simulink model "composition"  (R2024a)
settings: Solver=FixedStepDiscrete  StartTime=0.0  StopTime=10.0  RelTol=1e-3  EnableMultiTasking=on
undefined symbols (not defined in the file): D1, P
libraries: autosarlibdem x1, autosarlibnvm x1
settings Model: Creator=buiqu  LastModifiedBy=buiqu
settings SolverCC: AlgebraicLoopSolver=TrustRegion  AutoInsertRateTranBlk=on  InsertRTBMode=Never (minimum delay)  MaxZcPerStep=1
settings OptimizationCC: DefaultParameterBehavior=Inlined  EnhancedBackFolding=on  PassReuseOutputArgsAs=Individual arguments  ZeroExternalMemoryAtStartup=off  ZeroInternalMemoryAtStartup=off  OptimizeBlockOrder=speed  DifferentSizesBufferReuse=on  OptimizationCustomize=off  EfficientTunableParamExpr=on
settings DebuggingCC: MultiTaskDSMMsg=none  MultiTaskRateTransMsg=warning  ParameterTunabilityLossMsg=error  UnconnectedLineMsg=warning
settings ModelReferenceCC: EnableRefExpFcnMdlSchedulingChecks=on
settings SFSimCC: MATLABDynamicMemAlloc=off
settings RTWCC: Description=AUTOSAR  SystemTargetFile=autosar.tlc  GenCodeOnly=on  TemplateMakefile=ert_default_tmf  IncludeHyperlinkInReport=on  DataTypeReplacement=CDataTypesFixedWidth  GPUComputeCapability=3.5  DLArmComputeVersion=19.05
settings CodeAppCC: ForceParamTrailComments=on  IgnoreCustomStorageClasses=off  OperatorAnnotations=on  SimulinkDataObjDesc=on  SFDataObjDesc=on  InsertBlockDesc=on
settings STFCustomTargetCC: MultiwordLength=256  ParMdlRefBuildCompliant=on  CompOptLevelCompliant=on  IncludeMdlTerminateFcn=off  CombineOutputUpdateFcns=on  SuppressErrorStatus=on  ERTCustomFileBanners=on  SupportNonFinite=off  SupportComplex=off  SupportContinuousTime=off  SupportNonInlinedSFcns=off  RemoveResetFunc=on  MATLABClassNameForMDSCustomization=Simulink.SoftwareTarget.ERTCustomization  AutosarCompliant=on  GRTInterface=off  LookupTableObjectStructAxisOrder=2,1,3,4,...  LUTObjectStructOrderEvenSpacing=Size,Table,Breakpoints  SystemTargetFile=autosar.tlc
settings ERTTargetCC: TargetLangStandard=C99 (ISO)  ConcurrentExecutionCompliant=off  IncludeMdlTerminateFcn=off  SuppressErrorStatus=on  SupportNonFinite=off  SupportComplex=off  ModelStepFunctionPrototypeControlCompliant=off  CPPClassGenCompliant=off  AutosarCompliant=on  LookupTableObjectStructAxisOrder=2,1,3,4,...  LUTObjectStructOrderEvenSpacing=Size,Table,Breakpoints  InlinedParameterPlacement=NonHierarchical  ERTCustomFileTemplate=example_file_process.tlc  BooleanTrueId=TRUE  BooleanFalseId=FALSE

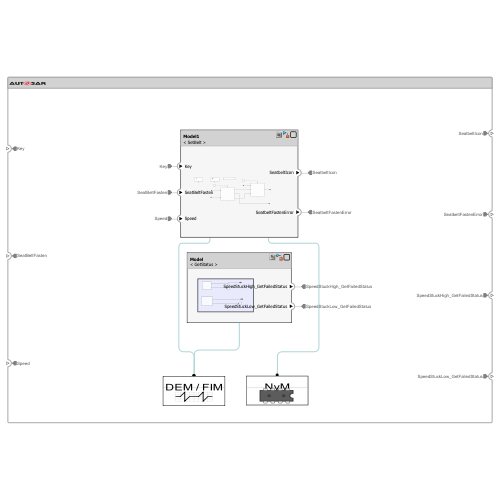
[thumbnail: Simulink's stored preview of the top-level diagram]
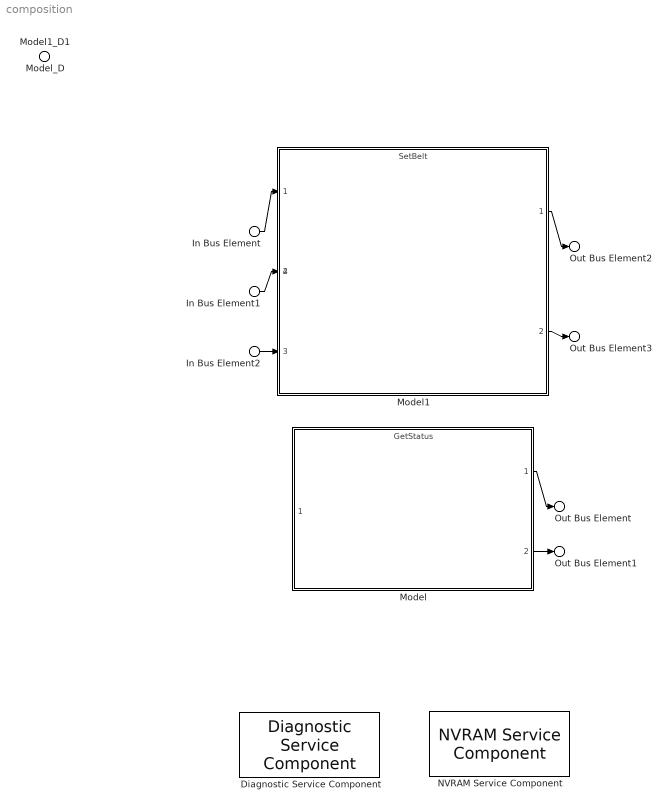
== system composition ==
  In Bus Element : Inport  PortName=Key
  In Bus Element1 : Inport  Port=2  PortName=SeatBeltFasten
  In Bus Element2 : Inport  Port=3  PortName=Speed
  Model_D : Inport  Port=4  OutputFunctionCall=on
  Model1_D1 : Inport  Port=5  OutputFunctionCall=on
  Diagnostic Service Component : autosarlibdem/Diagnostic Service Component  ClientPortNames={'SpeedStuckHigh', 'SpeedStuckLow'}  ClientPortPortDefinedArguments={'1', '2'}  MaxEventId=2  MaxFID=1  DemDebounceCounterIncrementStepSize=1  DemDebounceCounterDecrementStepSize=1  DemDebounceCounterFailedThreshold=2  DemDebounceCounterPassedThreshold=-1  InhibitionMatrix=[0 0;0 0]  EnableConditionIndexes=zeros(257,'uint8')  StorageConditionIndexes=zeros(257,'uint8')
  Model : ModelReference  ModelNameDialog=GetStatus  SimulationMode=Normal  ScheduleRates=on  CachedPortDiscreteRates=[-1]  ModelEventPortInfo=P:D1[-1][0][0]  CodeInterface=Top model  ModelReferenceVersion=1.12
      settings: PortSchema="{\"entries\":[{\"content\":{\"headerSize\":38,\"margin\":15,\"minimumSpacing\":25,\"sides\":[{\"content\":{},\"type\":\"ConnectorPlacement.EquallySpacedRectSide\",\"uuid\":\"70131014-7b1b-42d3-bc7e-7d162cdaf422\"},{\"content\":{\"connectorIds\":[\"Out1\",\"Out2\"],\"side\":\"RIGHT\"},\"type\":\"ConnectorPlacement.EquallySpacedRectSide\",\"uuid\":\"a8a66e78-9784-487d-a940-78f21da884fc\"},{\"content\":{\"side\":\"TOP\"},\"type\":\"ConnectorPlacement.EquallySpacedRectSide\",\"uuid\":\"0f6f6632-4e00-4b40-ae27-794534ba92f0\"},{\"content\":{\"connectorIds\":[\"In1\"],\"side\":\"HIDDEN\"},\"type\":\"ConnectorPlacement.EquallySpacedRectSide\",\"uuid\":\"c12b20b4-49c6-4eeb-a94e-0f049c51ebbe\"}]},\"type\":\"ConnectorPlacement.EquallySpacedConnector\",\"uuid\":\"080d5124-966e-4e64-be01-eaafe2cf5eb8\"}],\"packageUris\":[\"http://schema.mathworks.com/mf0/Connector/R2020b\"],\"version\":\"1.0\"}"
  Model1 : ModelReference  ModelNameDialog=SetBelt  SimulationMode=Normal  ScheduleRates=on  CachedPortDiscreteRates=[1]  ModelEventPortInfo=P:D1[1][0][0]  CodeInterface=Top model  ModelReferenceVersion=1.41
      settings: PortSchema="{\"entries\":[{\"content\":{\"headerSize\":38,\"margin\":15,\"minimumSpacing\":25,\"sides\":[{\"content\":{\"connectorIds\":[\"In1\",\"In2\",\"In3\"]},\"type\":\"ConnectorPlacement.EquallySpacedRectSide\",\"uuid\":\"70131014-7b1b-42d3-bc7e-7d162cdaf422\"},{\"content\":{\"connectorIds\":[\"Out1\",\"Out2\"],\"side\":\"RIGHT\"},\"type\":\"ConnectorPlacement.EquallySpacedRectSide\",\"uuid\":\"a8a66e78-9784-487d-a940-78f21da884fc\"},{\"content\":{\"side\":\"TOP\"},\"type\":\"ConnectorPlacement.EquallySpacedRectSide\",\"uuid\":\"0f6f6632-4e00-4b40-ae27-794534ba92f0\"},{\"content\":{\"connectorIds\":[\"In4\"],\"side\":\"HIDDEN\"},\"type\":\"ConnectorPlacement.EquallySpacedRectSide\",\"uuid\":\"93feeb0e-6d26-4a25-99a6-334197fb8ffe\"}]},\"type\":\"ConnectorPlacement.EquallySpacedConnector\",\"uuid\":\"080d5124-966e-4e64-be01-eaafe2cf5eb8\"}],\"packageUris\":[\"http://schema.mathworks.com/mf0/Connector/R2020b\"],\"version\":\"1.0\"}"
  NVRAM Service Component : autosarlibnvm/NVRAM Service Component  ClientPortNames={'IgnitionKeySwitchCount'}  ClientPortPortDefinedArguments={'1'}  MaxBlockId=10  NvInitValues={'0'}
  Out Bus Element2 : Outport  PortName=SeatbeltIcon
  Out Bus Element3 : Outport  Port=2  PortName=SeatbeltFastenError
  Out Bus Element : Outport  Port=3  PortName=SpeedStuckHigh_GetFailedStatus
  Out Bus Element1 : Outport  Port=4  PortName=SpeedStuckLow_GetFailedStatus
  wires:
  In Bus Element/1 -> Model1/1
  In Bus Element1/1 -> Model1/2
  In Bus Element2/1 -> Model1/3
  Model/1 -> Out Bus Element/1
  Model/2 -> Out Bus Element1/1
  Model1/1 -> Out Bus Element2/1
  Model1/2 -> Out Bus Element3/1
